simulink model "trial"  (R2016b)
settings: Solver=FixedStepDiscrete  StartTime=0  StopTime=9.8  FixedStep=0.2  RelTol=1e-3
values from neighbouring files (symbols this model uses):
  param_init_speed = 0    [init_workspace.m]
  param_N = 10    [init_workspace.m]
  param_R = 0    [init_workspace.m]
  param_ref_control = zeros(1,50)    [init_workspace.m]
  param_T = 0.2    [init_workspace.m]
undefined symbols (not defined in the file or in its folder): param_ref_speed
settings Model: Creator=mbatu  LastModifiedBy=mbatu

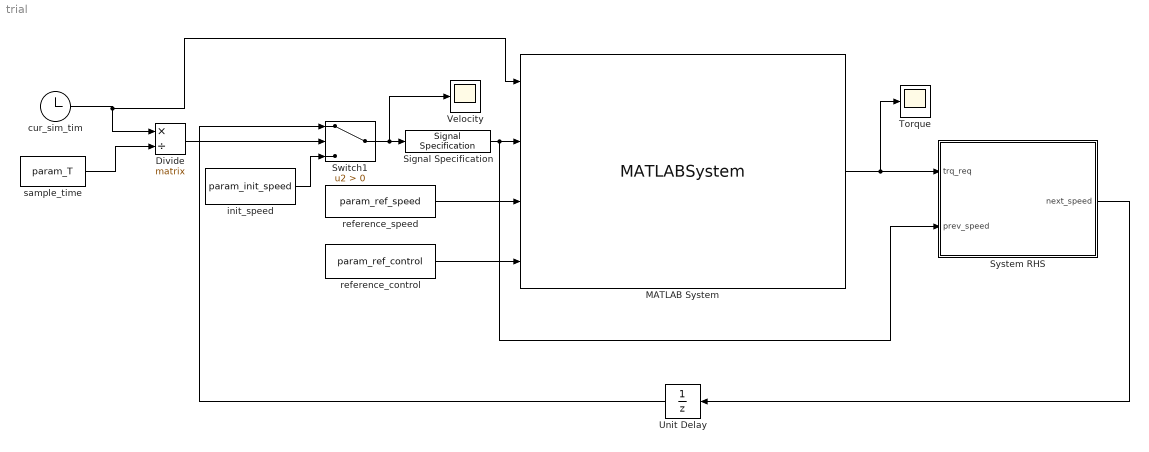
== system trial ==
  Divide : Product  Inputs=*/  Multiplication=Matrix(*)
  MATLAB System : MATLABSystem  System=MPC_Controller  T=param_T  N=param_N  Q=param_Q  R=param_R  Fbrake=param_Fbrake  Grade=param_Grade  SimulateUsing=Interpreted execution
      mask Type: MPC_Controller
      mask Display:
      | disp('MPC_Controller');
      | port_label('input',1,'cur_sim_tim');
      | port_label('input',2,'cur_speed');
      | port_label('input',3,'ref_speed');
      | port_label('input',4,'ref_control');
      | port_label('output',1,'trq_req');
  Signal Specification : SignalSpecification  OutDataTypeStr=double  Dimensions=[1,1]
  Switch1 : Switch  Criteria=u2 > Threshold
  System RHS : MATLAB Function  TreatAsAtomicUnit=on
  Torque : Scope
  Unit Delay : UnitDelay  SampleTime=-1
  Velocity : Scope
  cur_sim_tim : Clock
  init_speed : Constant  Value=param_init_speed
  reference_control : Constant  Value=param_ref_control
  reference_speed : Constant  Value=param_ref_speed  OutDataTypeStr=double
  sample_time : Constant  Value=param_T
  wires:
  cur_sim_tim/1 -> MATLAB System/1, Divide/1
  sample_time/1 -> Divide/2
  System RHS/1(next_speed) -> Unit Delay/1
  reference_speed/1 -> MATLAB System/3
  reference_control/1 -> MATLAB System/4
  MATLAB System/1 -> Torque/1, System RHS/1(trq_req)
  Divide/1 -> Switch1/2
  init_speed/1 -> Switch1/3
  Unit Delay/1 -> Switch1/1
  Signal Specification/1 -> System RHS/2(prev_speed), MATLAB System/2
  Switch1/1 -> Velocity/1, Signal Specification/1

== matlab function trial/System RHS ==
  data: trq_req input; prev_speed input; next_speed output
function next_speed = fcn(trq_req, prev_speed)

T = 0.2;           %sample time

% Constants for Vehicle Dynamics
Rtire  =  0.354;  % radius of tire(m)
G      =  9.81;   % earth's gravitational constant(m/s2)
mu     =  0.09;   % road friction(N) 
rho    =  1.225;  % density of air as a fluid(kg/m3)
Cd     =  0.55;   % air drag coefficient
A      =  5.1;    % vehicle frontal area(m2)
mss    =  2100;   % vehicle mass(kg)
ng     =  0.85;   % tire-specific constant
Im     =  0.18;   % motor inertia(kg*m2)
Gb     =  18.5;   % total gear ratio
 
% Variables for Vehicle Dynamics                                           
Fbrake    =  0;                             % braking force(N)
Grade     =  0;                             % grade(%)
alpha     =  atan(Grade/100);               % degree of slope(rad)
Faero     =  0.5*rho*A*Cd*(prev_speed^2);   % drag force against vehicle(N)
Frub      =  mu*mss*G;                      % rubbing force against tires(N)
Ftire     =  trq_req*Gb/Rtire;              % driving force(N)

dvdt      =  (Ftire - Frub - Faero - mss*G*sin(alpha) - Fbrake)/(mss + Im*Gb^2/(ng*Rtire^2));
next_speed = prev_speed + dvdt * T;
